simulink model "HIL5DOF_Speedgoat"  (R2026a)
settings: Solver=ode3  StopTime=inf  FixedStep=1/20000
values from neighbouring files (symbols this model uses):
  ems =     [ems11.mat]
  hems =     [Datos_Para_Control_Preciso.mat]
undefined symbols (not defined in the file or in its folder): hems_direct_F_table_H10, hems_direct_gap_bp_H10, hems_direct_I_bp_H10, IO316, IO3xx, m, magnitude, Pull, pull, up, x0, xguid_12, xguid_34, xguid_56, xlev_12, xlev_34, ylev_13, ylev_24, zguid
libraries: speedgoatlib_IO110 x2, aerolibobsolete x1, speedgoatlib_fpga_pwm x1, speedgoatlib_fpga x1
(part 2 of 2)

== system HIL5DOF_Speedgoat/MODELO ELECTROMAGNÉTICO/MODELO ELECTROMAGNETICO EMS/EMS 6 ==
  Tensión Objetivo : Inport
  Airgap : Inport  Port=2
  2-D Lookup Table1 : Lookup_n-D  BreakpointsForDimension1=ems.Airgap  BreakpointsForDimension2=ems.Current  Table=ems.Force_Horizontal  ExtrapMethod=Clip  InternalRulePriority=Speed  RndMeth=Simplest
      settings: InputPortMap=u0,u1
  CIrcuito RL : Subsystem
  Gain : Gain  Gain=1000
  Modelado Temperatura : Subsystem  Commented=through
  Corriente : Outport
  T [ºC] : Outport  Port=2
  Fuerza Horizontal : Outport  Port=3
  wires:
  CIrcuito RL/1(Corriente) -> 2-D Lookup Table1/2, Modelado Temperatura/1(I (A)), Corriente/1
  Tensión Objetivo/1 -> CIrcuito RL/2(Tensión Objetivo)
  Airgap/1 -> Gain/1, CIrcuito RL/1(Airgap)
  Gain/1 -> 2-D Lookup Table1/1
  Modelado Temperatura/1(T [ºC]) -> T [ºC]/1
  2-D Lookup Table1/1 -> Fuerza Horizontal/1

== system HIL5DOF_Speedgoat/MODELO ELECTROMAGNÉTICO/MODELO ELECTROMAGNETICO HEMS/HEMS 1 ==
  Tensión Objetivo : Inport
  Airgap : Inport  Port=2
  2-D Lookup Table1 : Lookup_n-D  Commented=on  BreakpointsForDimension1=hems.Airgap  BreakpointsForDimension2=hems.Current  Table=hems.Force_Horizontal  InternalRulePriority=Speed  RndMeth=Simplest
      settings: InputPortMap=u0,u1
  CIrcuito RL : Subsystem
  Gain : Gain  Gain=1000
  LUT_HEMS_1 : Lookup_n-D  BreakpointsForDimension1=hems_direct_gap_bp_H10  BreakpointsForDimension2=hems_direct_I_bp_H10  Table=hems_direct_F_table_H10  ExtrapMethod=Clip  InternalRulePriority=Speed  RndMeth=Simplest
      settings: InputPortMap=u0,u1
  Fuerza Vertical : Outport
  Corriente : Outport  Port=2
  Fuerza Horizontal : Outport  Port=3
  wires:
  CIrcuito RL/1(Corriente) -> LUT_HEMS_1/2, 2-D Lookup Table1/2, Corriente/1
  Tensión Objetivo/1 -> CIrcuito RL/2(Tensión Objetivo)
  LUT_HEMS_1/1 -> Fuerza Vertical/1
  Airgap/1 -> Gain/1, CIrcuito RL/1(Airgap)
  Gain/1 -> LUT_HEMS_1/1, 2-D Lookup Table1/1
  2-D Lookup Table1/1 -> Fuerza Horizontal/1

== system HIL5DOF_Speedgoat/MODELO ELECTROMAGNÉTICO/MODELO ELECTROMAGNETICO HEMS/HEMS 2 ==
  Tensión Objetivo : Inport
  Airgap : Inport  Port=2
  2-D Lookup Table1 : Lookup_n-D  Commented=on  BreakpointsForDimension1=hems.Airgap  BreakpointsForDimension2=hems.Current  Table=hems.Force_Horizontal  InternalRulePriority=Speed  RndMeth=Simplest
      settings: InputPortMap=u0,u1
  CIrcuito RL : Subsystem
  Gain : Gain  Gain=1000
  LUT_HEMS_1 : Lookup_n-D  BreakpointsForDimension1=hems_direct_gap_bp_H10  BreakpointsForDimension2=hems_direct_I_bp_H10  Table=hems_direct_F_table_H10  ExtrapMethod=Clip  InternalRulePriority=Speed  RndMeth=Simplest
      settings: InputPortMap=u0,u1
  Modelado Temperatura : Subsystem
  Fuerza Vertical : Outport
  Corriente : Outport  Port=2
  T [ºC] : Outport  Port=3
  Fuerza Horizontal : Outport  Port=4
  wires:
  2-D Lookup Table1/1 -> Fuerza Horizontal/1
  Modelado Temperatura/1(T [ºC]) -> T [ºC]/1
  Gain/1 -> LUT_HEMS_1/1, 2-D Lookup Table1/1
  Airgap/1 -> CIrcuito RL/1(Airgap), Gain/1
  LUT_HEMS_1/1 -> Fuerza Vertical/1
  Tensión Objetivo/1 -> CIrcuito RL/2(Tensión Objetivo)
  CIrcuito RL/1(Corriente) -> Corriente/1, LUT_HEMS_1/2, Modelado Temperatura/1(I (A)), 2-D Lookup Table1/2

== system HIL5DOF_Speedgoat/MODELO ELECTROMAGNÉTICO/MODELO ELECTROMAGNETICO HEMS/HEMS 3 ==
  Tensión Objetivo : Inport
  Airgap : Inport  Port=2
  2-D Lookup Table1 : Lookup_n-D  Commented=on  BreakpointsForDimension1=hems.Airgap  BreakpointsForDimension2=hems.Current  Table=hems.Force_Horizontal  InternalRulePriority=Speed  RndMeth=Simplest
      settings: InputPortMap=u0,u1
  CIrcuito RL : Subsystem
  Gain : Gain  Gain=1000
  LUT_HEMS_1 : Lookup_n-D  BreakpointsForDimension1=hems_direct_gap_bp_H10  BreakpointsForDimension2=hems_direct_I_bp_H10  Table=hems_direct_F_table_H10  ExtrapMethod=Clip  InternalRulePriority=Speed  RndMeth=Simplest
      settings: InputPortMap=u0,u1
  Modelado Temperatura : Subsystem
  Fuerza Vertical : Outport
  Corriente : Outport  Port=2
  T [ºC] : Outport  Port=3
  Fuerza Horizontal : Outport  Port=4
  wires:
  CIrcuito RL/1(Corriente) -> LUT_HEMS_1/2, 2-D Lookup Table1/2, Modelado Temperatura/1(I (A)), Corriente/1
  Tensión Objetivo/1 -> CIrcuito RL/2(Tensión Objetivo)
  LUT_HEMS_1/1 -> Fuerza Vertical/1
  Airgap/1 -> Gain/1, CIrcuito RL/1(Airgap)
  Gain/1 -> LUT_HEMS_1/1, 2-D Lookup Table1/1
  Modelado Temperatura/1(T [ºC]) -> T [ºC]/1
  2-D Lookup Table1/1 -> Fuerza Horizontal/1

== system HIL5DOF_Speedgoat/MODELO ELECTROMAGNÉTICO/MODELO ELECTROMAGNETICO HEMS/HEMS 4 ==
  Tensión Objetivo : Inport
  Airgap : Inport  Port=2
  2-D Lookup Table1 : Lookup_n-D  Commented=on  BreakpointsForDimension1=hems.Airgap  BreakpointsForDimension2=hems.Current  Table=hems.Force_Horizontal  InternalRulePriority=Speed  RndMeth=Simplest
      settings: InputPortMap=u0,u1
  CIrcuito RL : Subsystem
  Gain : Gain  Gain=1000
  LUT_HEMS_1 : Lookup_n-D  BreakpointsForDimension1=hems_direct_gap_bp_H10  BreakpointsForDimension2=hems_direct_I_bp_H10  Table=hems_direct_F_table_H10  ExtrapMethod=Clip  InternalRulePriority=Speed  RndMeth=Simplest
      settings: InputPortMap=u0,u1
  Modelado Temperatura : Subsystem
  Fuerza Vertical : Outport
  Corriente : Outport  Port=2
  T [ºC] : Outport  Port=3
  Fuerza Horizontal : Outport  Port=4
  wires:
  2-D Lookup Table1/1 -> Fuerza Horizontal/1
  Modelado Temperatura/1(T [ºC]) -> T [ºC]/1
  Gain/1 -> LUT_HEMS_1/1, 2-D Lookup Table1/1
  Airgap/1 -> CIrcuito RL/1(Airgap), Gain/1
  LUT_HEMS_1/1 -> Fuerza Vertical/1
  Tensión Objetivo/1 -> CIrcuito RL/2(Tensión Objetivo)
  CIrcuito RL/1(Corriente) -> Corriente/1, LUT_HEMS_1/2, Modelado Temperatura/1(I (A)), 2-D Lookup Table1/2

== system HIL5DOF_Speedgoat/MODELO ELECTROMAGNÉTICO/MODELO ELECTROMAGNETICO EMS/EMS 1/CIrcuito RL ==
  Airgap : Inport
  Tensión Objetivo : Inport  Port=2
  Add : Sum  Inputs=+-
  Gain : Gain  Gain=1000
  Inductancia de la Bobina : Lookup_n-D  BreakpointsForDimension1=ems.Airgap  BreakpointsForDimension2=ems.Current(1:54)  Table=ems.Inductance  ExtrapMethod=Clip  InternalRulePriority=Speed  RndMeth=Simplest
      settings: InputPortMap=u0,u1
  Integrator : Integrator
  Product : Product  Inputs=*/
  Product1 : Product  Inputs=/*
  Product2 : Product  Inputs=*/
  Resistencia : Constant  Value=hems.Resistance
  Corriente : Outport
  wires:
  Gain/1 -> Inductancia de la Bobina/1
  Tensión Objetivo/1 -> Product/1
  Product2/1 -> Integrator/1
  Add/1 -> Product2/1
  Integrator/1 -> Add/2, Inductancia de la Bobina/2, Corriente/1
  Airgap/1 -> Gain/1
  Resistencia/1 -> Product/2, Product1/1
  Product/1 -> Add/1
  Product1/1 -> Product2/2
  Inductancia de la Bobina/1 -> Product1/2

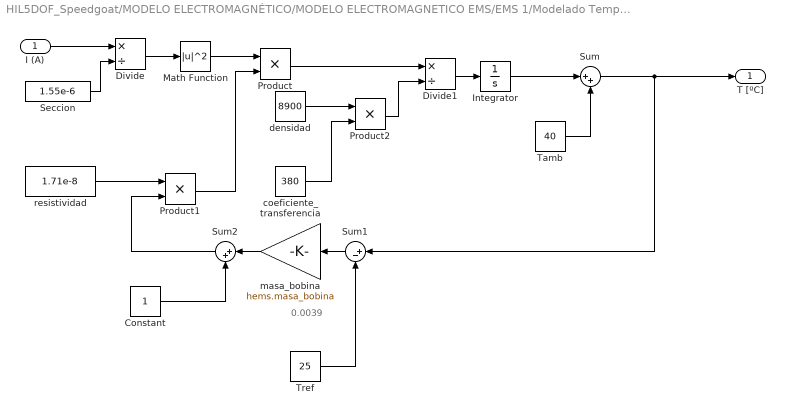
== system HIL5DOF_Speedgoat/MODELO ELECTROMAGNÉTICO/MODELO ELECTROMAGNETICO EMS/EMS 1/Modelado Temperatura ==
  note: 0.0039
  I (A) : Inport
  Constant : Constant
  Divide : Product  Inputs=*/
  Divide1 : Product  Inputs=*/
  Integrator : Integrator
  Math Function : Math  Operator=magnitude^2
  Product : Product
  Product1 : Product
  Product2 : Product
  Seccion : Constant  Value=1.55e-6
  Sum : Sum  Inputs=|++
  Sum1 : Sum  Inputs=|+-
  Sum2 : Sum  Inputs=|++
  Tamb : Constant  Value=40
  Tref : Constant  Value=25
  coeficiente_transferencia : Constant  Value=380
  densidad : Constant  Value=8900
  masa_bobina : Gain  Gain=hems.masa_bobina
  resistividad : Constant  Value=1.71e-8
  T [ºC] : Outport
  wires:
  I (A)/1 -> Divide/1
  Product2/1 -> Divide1/2
  Tref/1 -> Sum1/2
  Tamb/1 -> Sum/2
  Product/1 -> Divide1/1
  masa_bobina/1 -> Sum2/1
  coeficiente_transferencia/1 -> Product2/2
  Sum2/1 -> Product1/2
  Math Function/1 -> Product/1
  Sum/1 -> Sum1/1, T [ºC]/1
  Product1/1 -> Product/2
  Constant/1 -> Sum2/2
  resistividad/1 -> Product1/1
  Divide/1 -> Math Function/1
  densidad/1 -> Product2/1
  Divide1/1 -> Integrator/1
  Seccion/1 -> Divide/2
  Sum1/1 -> masa_bobina/1
  Integrator/1 -> Sum/1

== system HIL5DOF_Speedgoat/MODELO ELECTROMAGNÉTICO/MODELO ELECTROMAGNETICO EMS/EMS 2/CIrcuito RL ==
  Airgap : Inport
  Tensión Objetivo : Inport  Port=2
  Add : Sum  Inputs=+-
  Gain : Gain  Gain=1000
  Inductancia de la Bobina : Lookup_n-D  BreakpointsForDimension1=ems.Airgap  BreakpointsForDimension2=ems.Current(1:54)  Table=ems.Inductance  ExtrapMethod=Clip  InternalRulePriority=Speed  RndMeth=Simplest
      settings: InputPortMap=u0,u1
  Integrator : Integrator
  Product : Product  Inputs=*/
  Product1 : Product  Inputs=/*
  Product2 : Product  Inputs=*/
  Resistencia : Constant  Value=hems.Resistance
  Corriente : Outport
  wires:
  Inductancia de la Bobina/1 -> Product1/2
  Product1/1 -> Product2/2
  Product/1 -> Add/1
  Resistencia/1 -> Product1/1, Product/2
  Airgap/1 -> Gain/1
  Integrator/1 -> Corriente/1, Inductancia de la Bobina/2, Add/2
  Add/1 -> Product2/1
  Product2/1 -> Integrator/1
  Tensión Objetivo/1 -> Product/1
  Gain/1 -> Inductancia de la Bobina/1

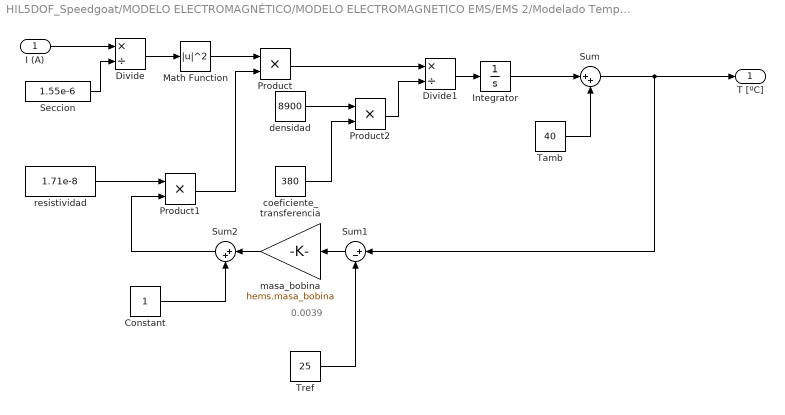
== system HIL5DOF_Speedgoat/MODELO ELECTROMAGNÉTICO/MODELO ELECTROMAGNETICO EMS/EMS 2/Modelado Temperatura ==
  note: 0.0039
  I (A) : Inport
  Constant : Constant
  Divide : Product  Inputs=*/
  Divide1 : Product  Inputs=*/
  Integrator : Integrator
  Math Function : Math  Operator=magnitude^2
  Product : Product
  Product1 : Product
  Product2 : Product
  Seccion : Constant  Value=1.55e-6
  Sum : Sum  Inputs=|++
  Sum1 : Sum  Inputs=|+-
  Sum2 : Sum  Inputs=|++
  Tamb : Constant  Value=40
  Tref : Constant  Value=25
  coeficiente_transferencia : Constant  Value=380
  densidad : Constant  Value=8900
  masa_bobina : Gain  Gain=hems.masa_bobina
  resistividad : Constant  Value=1.71e-8
  T [ºC] : Outport
  wires:
  Integrator/1 -> Sum/1
  Sum1/1 -> masa_bobina/1
  Seccion/1 -> Divide/2
  Divide1/1 -> Integrator/1
  densidad/1 -> Product2/1
  Divide/1 -> Math Function/1
  resistividad/1 -> Product1/1
  Constant/1 -> Sum2/2
  Product1/1 -> Product/2
  Sum/1 -> T [ºC]/1, Sum1/1
  Math Function/1 -> Product/1
  Sum2/1 -> Product1/2
  coeficiente_transferencia/1 -> Product2/2
  masa_bobina/1 -> Sum2/1
  Product/1 -> Divide1/1
  Tamb/1 -> Sum/2
  Tref/1 -> Sum1/2
  Product2/1 -> Divide1/2
  I (A)/1 -> Divide/1

== system HIL5DOF_Speedgoat/MODELO ELECTROMAGNÉTICO/MODELO ELECTROMAGNETICO EMS/EMS 3/CIrcuito RL ==
  Airgap : Inport
  Tensión Objetivo : Inport  Port=2
  Add : Sum  Inputs=+-
  Gain : Gain  Gain=1000
  Inductancia de la Bobina : Lookup_n-D  BreakpointsForDimension1=ems.Airgap  BreakpointsForDimension2=ems.Current(1:54)  Table=ems.Inductance  ExtrapMethod=Clip  InternalRulePriority=Speed  RndMeth=Simplest
      settings: InputPortMap=u0,u1
  Integrator : Integrator
  Product : Product  Inputs=*/
  Product1 : Product  Inputs=/*
  Product2 : Product  Inputs=*/
  Resistencia : Constant  Value=hems.Resistance
  Corriente : Outport
  wires:
  Gain/1 -> Inductancia de la Bobina/1
  Tensión Objetivo/1 -> Product/1
  Product2/1 -> Integrator/1
  Add/1 -> Product2/1
  Integrator/1 -> Add/2, Inductancia de la Bobina/2, Corriente/1
  Airgap/1 -> Gain/1
  Resistencia/1 -> Product/2, Product1/1
  Product/1 -> Add/1
  Product1/1 -> Product2/2
  Inductancia de la Bobina/1 -> Product1/2

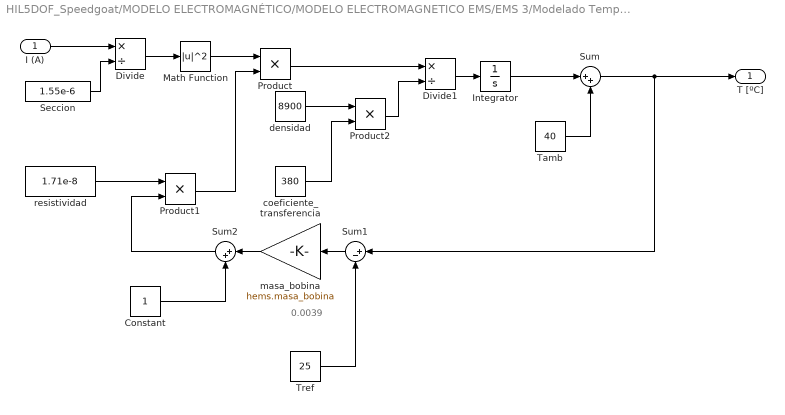
== system HIL5DOF_Speedgoat/MODELO ELECTROMAGNÉTICO/MODELO ELECTROMAGNETICO EMS/EMS 3/Modelado Temperatura ==
  note: 0.0039
  I (A) : Inport
  Constant : Constant
  Divide : Product  Inputs=*/
  Divide1 : Product  Inputs=*/
  Integrator : Integrator
  Math Function : Math  Operator=magnitude^2
  Product : Product
  Product1 : Product
  Product2 : Product
  Seccion : Constant  Value=1.55e-6
  Sum : Sum  Inputs=|++
  Sum1 : Sum  Inputs=|+-
  Sum2 : Sum  Inputs=|++
  Tamb : Constant  Value=40
  Tref : Constant  Value=25
  coeficiente_transferencia : Constant  Value=380
  densidad : Constant  Value=8900
  masa_bobina : Gain  Gain=hems.masa_bobina
  resistividad : Constant  Value=1.71e-8
  T [ºC] : Outport
  wires:
  I (A)/1 -> Divide/1
  Product2/1 -> Divide1/2
  Tref/1 -> Sum1/2
  Tamb/1 -> Sum/2
  Product/1 -> Divide1/1
  masa_bobina/1 -> Sum2/1
  coeficiente_transferencia/1 -> Product2/2
  Sum2/1 -> Product1/2
  Math Function/1 -> Product/1
  Sum/1 -> Sum1/1, T [ºC]/1
  Product1/1 -> Product/2
  Constant/1 -> Sum2/2
  resistividad/1 -> Product1/1
  Divide/1 -> Math Function/1
  densidad/1 -> Product2/1
  Divide1/1 -> Integrator/1
  Seccion/1 -> Divide/2
  Sum1/1 -> masa_bobina/1
  Integrator/1 -> Sum/1

== system HIL5DOF_Speedgoat/MODELO ELECTROMAGNÉTICO/MODELO ELECTROMAGNETICO EMS/EMS 4/CIrcuito RL ==
  Airgap : Inport
  Tensión Objetivo : Inport  Port=2
  Add : Sum  Inputs=+-
  Gain : Gain  Gain=1000
  Inductancia de la Bobina : Lookup_n-D  BreakpointsForDimension1=ems.Airgap  BreakpointsForDimension2=ems.Current(1:54)  Table=ems.Inductance  ExtrapMethod=Clip  InternalRulePriority=Speed  RndMeth=Simplest
      settings: InputPortMap=u0,u1
  Integrator : Integrator
  Product : Product  Inputs=*/
  Product1 : Product  Inputs=/*
  Product2 : Product  Inputs=*/
  Resistencia : Constant  Value=hems.Resistance
  Corriente : Outport
  wires:
  Inductancia de la Bobina/1 -> Product1/2
  Product1/1 -> Product2/2
  Product/1 -> Add/1
  Resistencia/1 -> Product1/1, Product/2
  Airgap/1 -> Gain/1
  Integrator/1 -> Corriente/1, Inductancia de la Bobina/2, Add/2
  Add/1 -> Product2/1
  Product2/1 -> Integrator/1
  Tensión Objetivo/1 -> Product/1
  Gain/1 -> Inductancia de la Bobina/1

== system HIL5DOF_Speedgoat/MODELO ELECTROMAGNÉTICO/MODELO ELECTROMAGNETICO EMS/EMS 4/Modelado Temperatura ==
  note: 0.0039
  I (A) : Inport
  Constant : Constant
  Divide : Product  Inputs=*/
  Divide1 : Product  Inputs=*/
  Integrator : Integrator
  Math Function : Math  Operator=magnitude^2
  Product : Product
  Product1 : Product
  Product2 : Product
  Seccion : Constant  Value=1.55e-6
  Sum : Sum  Inputs=|++
  Sum1 : Sum  Inputs=|+-
  Sum2 : Sum  Inputs=|++
  Tamb : Constant  Value=40
  Tref : Constant  Value=25
  coeficiente_transferencia : Constant  Value=380
  densidad : Constant  Value=8900
  masa_bobina : Gain  Gain=hems.masa_bobina
  resistividad : Constant  Value=1.71e-8
  T [ºC] : Outport
  wires:
  Integrator/1 -> Sum/1
  Sum1/1 -> masa_bobina/1
  Seccion/1 -> Divide/2
  Divide1/1 -> Integrator/1
  densidad/1 -> Product2/1
  Divide/1 -> Math Function/1
  resistividad/1 -> Product1/1
  Constant/1 -> Sum2/2
  Product1/1 -> Product/2
  Sum/1 -> T [ºC]/1, Sum1/1
  Math Function/1 -> Product/1
  Sum2/1 -> Product1/2
  coeficiente_transferencia/1 -> Product2/2
  masa_bobina/1 -> Sum2/1
  Product/1 -> Divide1/1
  Tamb/1 -> Sum/2
  Tref/1 -> Sum1/2
  Product2/1 -> Divide1/2
  I (A)/1 -> Divide/1

== system HIL5DOF_Speedgoat/MODELO ELECTROMAGNÉTICO/MODELO ELECTROMAGNETICO EMS/EMS 5/CIrcuito RL ==
  Airgap : Inport
  Tensión Objetivo : Inport  Port=2
  Add : Sum  Inputs=+-
  Gain : Gain  Gain=1000
  Inductancia de la Bobina : Lookup_n-D  BreakpointsForDimension1=ems.Airgap  BreakpointsForDimension2=ems.Current(1:54)  Table=ems.Inductance  ExtrapMethod=Clip  InternalRulePriority=Speed  RndMeth=Simplest
      settings: InputPortMap=u0,u1
  Integrator : Integrator
  Product : Product  Inputs=*/
  Product1 : Product  Inputs=/*
  Product2 : Product  Inputs=*/
  Resistencia : Constant  Value=hems.Resistance
  Corriente : Outport
  wires:
  Gain/1 -> Inductancia de la Bobina/1
  Tensión Objetivo/1 -> Product/1
  Product2/1 -> Integrator/1
  Add/1 -> Product2/1
  Integrator/1 -> Add/2, Inductancia de la Bobina/2, Corriente/1
  Airgap/1 -> Gain/1
  Resistencia/1 -> Product/2, Product1/1
  Product/1 -> Add/1
  Product1/1 -> Product2/2
  Inductancia de la Bobina/1 -> Product1/2

== system HIL5DOF_Speedgoat/MODELO ELECTROMAGNÉTICO/MODELO ELECTROMAGNETICO EMS/EMS 5/Modelado Temperatura ==
  note: 0.0039
  I (A) : Inport
  Constant : Constant
  Divide : Product  Inputs=*/
  Divide1 : Product  Inputs=*/
  Integrator : Integrator
  Math Function : Math  Operator=magnitude^2
  Product : Product
  Product1 : Product
  Product2 : Product
  Seccion : Constant  Value=1.55e-6
  Sum : Sum  Inputs=|++
  Sum1 : Sum  Inputs=|+-
  Sum2 : Sum  Inputs=|++
  Tamb : Constant  Value=40
  Tref : Constant  Value=25
  coeficiente_transferencia : Constant  Value=380
  densidad : Constant  Value=8900
  masa_bobina : Gain  Gain=hems.masa_bobina
  resistividad : Constant  Value=1.71e-8
  T [ºC] : Outport
  wires:
  I (A)/1 -> Divide/1
  Product2/1 -> Divide1/2
  Tref/1 -> Sum1/2
  Tamb/1 -> Sum/2
  Product/1 -> Divide1/1
  masa_bobina/1 -> Sum2/1
  coeficiente_transferencia/1 -> Product2/2
  Sum2/1 -> Product1/2
  Math Function/1 -> Product/1
  Sum/1 -> Sum1/1, T [ºC]/1
  Product1/1 -> Product/2
  Constant/1 -> Sum2/2
  resistividad/1 -> Product1/1
  Divide/1 -> Math Function/1
  densidad/1 -> Product2/1
  Divide1/1 -> Integrator/1
  Seccion/1 -> Divide/2
  Sum1/1 -> masa_bobina/1
  Integrator/1 -> Sum/1

== system HIL5DOF_Speedgoat/MODELO ELECTROMAGNÉTICO/MODELO ELECTROMAGNETICO EMS/EMS 6/CIrcuito RL ==
  Airgap : Inport
  Tensión Objetivo : Inport  Port=2
  Add : Sum  Inputs=+-
  Gain : Gain  Gain=1000
  Inductancia de la Bobina : Lookup_n-D  BreakpointsForDimension1=ems.Airgap  BreakpointsForDimension2=ems.Current(1:54)  Table=ems.Inductance  ExtrapMethod=Clip  InternalRulePriority=Speed  RndMeth=Simplest
      settings: InputPortMap=u0,u1
  Integrator : Integrator
  Product : Product  Inputs=*/
  Product1 : Product  Inputs=/*
  Product2 : Product  Inputs=*/
  Resistencia : Constant  Value=hems.Resistance
  Corriente : Outport
  wires:
  Inductancia de la Bobina/1 -> Product1/2
  Product1/1 -> Product2/2
  Product/1 -> Add/1
  Resistencia/1 -> Product1/1, Product/2
  Airgap/1 -> Gain/1
  Integrator/1 -> Corriente/1, Inductancia de la Bobina/2, Add/2
  Add/1 -> Product2/1
  Product2/1 -> Integrator/1
  Tensión Objetivo/1 -> Product/1
  Gain/1 -> Inductancia de la Bobina/1

== system HIL5DOF_Speedgoat/MODELO ELECTROMAGNÉTICO/MODELO ELECTROMAGNETICO EMS/EMS 6/Modelado Temperatura ==
  note: 0.0039
  I (A) : Inport
  Constant : Constant
  Divide : Product  Inputs=*/
  Divide1 : Product  Inputs=*/
  Integrator : Integrator
  Math Function : Math  Operator=magnitude^2
  Product : Product
  Product1 : Product
  Product2 : Product
  Seccion : Constant  Value=1.55e-6
  Sum : Sum  Inputs=|++
  Sum1 : Sum  Inputs=|+-
  Sum2 : Sum  Inputs=|++
  Tamb : Constant  Value=40
  Tref : Constant  Value=25
  coeficiente_transferencia : Constant  Value=380
  densidad : Constant  Value=8900
  masa_bobina : Gain  Gain=hems.masa_bobina
  resistividad : Constant  Value=1.71e-8
  T [ºC] : Outport
  wires:
  Integrator/1 -> Sum/1
  Sum1/1 -> masa_bobina/1
  Seccion/1 -> Divide/2
  Divide1/1 -> Integrator/1
  densidad/1 -> Product2/1
  Divide/1 -> Math Function/1
  resistividad/1 -> Product1/1
  Constant/1 -> Sum2/2
  Product1/1 -> Product/2
  Sum/1 -> T [ºC]/1, Sum1/1
  Math Function/1 -> Product/1
  Sum2/1 -> Product1/2
  coeficiente_transferencia/1 -> Product2/2
  masa_bobina/1 -> Sum2/1
  Product/1 -> Divide1/1
  Tamb/1 -> Sum/2
  Tref/1 -> Sum1/2
  Product2/1 -> Divide1/2
  I (A)/1 -> Divide/1

== system HIL5DOF_Speedgoat/MODELO ELECTROMAGNÉTICO/MODELO ELECTROMAGNETICO HEMS/HEMS 1/CIrcuito RL ==
  Airgap : Inport
  Tensión Objetivo : Inport  Port=2
  Add : Sum  Inputs=+-
  Gain : Gain  Gain=1000
  Inductancia de la Bobina : Lookup_n-D  BreakpointsForDimension1=hems.Airgap  BreakpointsForDimension2=hems.Current(1:109)  Table=hems.Inductance  InternalRulePriority=Speed  RndMeth=Simplest
      settings: InputPortMap=u0,u1
  Integrator : Integrator
  Product : Product  Inputs=*/
  Product1 : Product  Inputs=/*
  Product2 : Product  Inputs=*/
  Resistencia : Constant  Value=hems.Resistance
  Corriente : Outport
  wires:
  Inductancia de la Bobina/1 -> Product1/2
  Product1/1 -> Product2/2
  Product/1 -> Add/1
  Resistencia/1 -> Product1/1, Product/2
  Airgap/1 -> Gain/1
  Integrator/1 -> Corriente/1, Inductancia de la Bobina/2, Add/2
  Add/1 -> Product2/1
  Product2/1 -> Integrator/1
  Tensión Objetivo/1 -> Product/1
  Gain/1 -> Inductancia de la Bobina/1

== system HIL5DOF_Speedgoat/MODELO ELECTROMAGNÉTICO/MODELO ELECTROMAGNETICO HEMS/HEMS 2/CIrcuito RL ==
  Airgap : Inport
  Tensión Objetivo : Inport  Port=2
  Add : Sum  Inputs=+-
  Gain : Gain  Gain=1000
  Inductancia de la Bobina : Lookup_n-D  BreakpointsForDimension1=hems.Airgap  BreakpointsForDimension2=hems.Current(1:109)  Table=hems.Inductance  InternalRulePriority=Speed  RndMeth=Simplest
      settings: InputPortMap=u0,u1
  Integrator : Integrator
  Product : Product  Inputs=*/
  Product1 : Product  Inputs=/*
  Product2 : Product  Inputs=*/
  Resistencia : Constant  Value=hems.Resistance
  Corriente : Outport
  wires:
  Gain/1 -> Inductancia de la Bobina/1
  Tensión Objetivo/1 -> Product/1
  Product2/1 -> Integrator/1
  Add/1 -> Product2/1
  Integrator/1 -> Add/2, Inductancia de la Bobina/2, Corriente/1
  Airgap/1 -> Gain/1
  Resistencia/1 -> Product/2, Product1/1
  Product/1 -> Add/1
  Product1/1 -> Product2/2
  Inductancia de la Bobina/1 -> Product1/2

== system HIL5DOF_Speedgoat/MODELO ELECTROMAGNÉTICO/MODELO ELECTROMAGNETICO HEMS/HEMS 2/Modelado Temperatura ==
  note: 0.0039
  I (A) : Inport
  Constant : Constant
  Divide : Product  Inputs=*/
  Divide1 : Product  Inputs=*/
  Integrator : Integrator
  Math Function : Math  Operator=magnitude^2
  Product : Product
  Product1 : Product
  Product2 : Product
  Seccion : Constant  Value=1.55e-6
  Sum : Sum  Inputs=|++
  Sum1 : Sum  Inputs=|+-
  Sum2 : Sum  Inputs=|++
  Tamb : Constant  Value=40
  Tref : Constant  Value=25
  coeficiente_transferencia : Constant  Value=380
  densidad : Constant  Value=8900
  masa_bobina : Gain  Gain=hems.masa_bobina
  resistividad : Constant  Value=1.71e-8
  T [ºC] : Outport
  wires:
  I (A)/1 -> Divide/1
  Product2/1 -> Divide1/2
  Tref/1 -> Sum1/2
  Tamb/1 -> Sum/2
  Product/1 -> Divide1/1
  masa_bobina/1 -> Sum2/1
  coeficiente_transferencia/1 -> Product2/2
  Sum2/1 -> Product1/2
  Math Function/1 -> Product/1
  Sum/1 -> Sum1/1, T [ºC]/1
  Product1/1 -> Product/2
  Constant/1 -> Sum2/2
  resistividad/1 -> Product1/1
  Divide/1 -> Math Function/1
  densidad/1 -> Product2/1
  Divide1/1 -> Integrator/1
  Seccion/1 -> Divide/2
  Sum1/1 -> masa_bobina/1
  Integrator/1 -> Sum/1

== system HIL5DOF_Speedgoat/MODELO ELECTROMAGNÉTICO/MODELO ELECTROMAGNETICO HEMS/HEMS 3/CIrcuito RL ==
  Airgap : Inport
  Tensión Objetivo : Inport  Port=2
  Add : Sum  Inputs=+-
  Gain : Gain  Gain=1000
  Inductancia de la Bobina : Lookup_n-D  BreakpointsForDimension1=hems.Airgap  BreakpointsForDimension2=hems.Current(1:109)  Table=hems.Inductance  InternalRulePriority=Speed  RndMeth=Simplest
      settings: InputPortMap=u0,u1
  Integrator : Integrator
  Product : Product  Inputs=*/
  Product1 : Product  Inputs=/*
  Product2 : Product  Inputs=*/
  Resistencia : Constant  Value=hems.Resistance
  Corriente : Outport
  wires:
  Inductancia de la Bobina/1 -> Product1/2
  Product1/1 -> Product2/2
  Product/1 -> Add/1
  Resistencia/1 -> Product1/1, Product/2
  Airgap/1 -> Gain/1
  Integrator/1 -> Corriente/1, Inductancia de la Bobina/2, Add/2
  Add/1 -> Product2/1
  Product2/1 -> Integrator/1
  Tensión Objetivo/1 -> Product/1
  Gain/1 -> Inductancia de la Bobina/1

== system HIL5DOF_Speedgoat/MODELO ELECTROMAGNÉTICO/MODELO ELECTROMAGNETICO HEMS/HEMS 3/Modelado Temperatura ==
  note: 0.0039
  I (A) : Inport
  Constant : Constant
  Divide : Product  Inputs=*/
  Divide1 : Product  Inputs=*/
  Integrator : Integrator
  Math Function : Math  Operator=magnitude^2
  Product : Product
  Product1 : Product
  Product2 : Product
  Seccion : Constant  Value=1.55e-6
  Sum : Sum  Inputs=|++
  Sum1 : Sum  Inputs=|+-
  Sum2 : Sum  Inputs=|++
  Tamb : Constant  Value=40
  Tref : Constant  Value=25
  coeficiente_transferencia : Constant  Value=380
  densidad : Constant  Value=8900
  masa_bobina : Gain  Gain=hems.masa_bobina
  resistividad : Constant  Value=1.71e-8
  T [ºC] : Outport
  wires:
  Integrator/1 -> Sum/1
  Sum1/1 -> masa_bobina/1
  Seccion/1 -> Divide/2
  Divide1/1 -> Integrator/1
  densidad/1 -> Product2/1
  Divide/1 -> Math Function/1
  resistividad/1 -> Product1/1
  Constant/1 -> Sum2/2
  Product1/1 -> Product/2
  Sum/1 -> T [ºC]/1, Sum1/1
  Math Function/1 -> Product/1
  Sum2/1 -> Product1/2
  coeficiente_transferencia/1 -> Product2/2
  masa_bobina/1 -> Sum2/1
  Product/1 -> Divide1/1
  Tamb/1 -> Sum/2
  Tref/1 -> Sum1/2
  Product2/1 -> Divide1/2
  I (A)/1 -> Divide/1

== system HIL5DOF_Speedgoat/MODELO ELECTROMAGNÉTICO/MODELO ELECTROMAGNETICO HEMS/HEMS 4/CIrcuito RL ==
  Airgap : Inport
  Tensión Objetivo : Inport  Port=2
  Add : Sum  Inputs=+-
  Gain : Gain  Gain=1000
  Inductancia de la Bobina : Lookup_n-D  BreakpointsForDimension1=hems.Airgap  BreakpointsForDimension2=hems.Current(1:109)  Table=hems.Inductance  InternalRulePriority=Speed  RndMeth=Simplest
      settings: InputPortMap=u0,u1
  Integrator : Integrator
  Product : Product  Inputs=*/
  Product1 : Product  Inputs=/*
  Product2 : Product  Inputs=*/
  Resistencia : Constant  Value=hems.Resistance
  Corriente : Outport
  wires:
  Gain/1 -> Inductancia de la Bobina/1
  Tensión Objetivo/1 -> Product/1
  Product2/1 -> Integrator/1
  Add/1 -> Product2/1
  Integrator/1 -> Add/2, Inductancia de la Bobina/2, Corriente/1
  Airgap/1 -> Gain/1
  Resistencia/1 -> Product/2, Product1/1
  Product/1 -> Add/1
  Product1/1 -> Product2/2
  Inductancia de la Bobina/1 -> Product1/2

== system HIL5DOF_Speedgoat/MODELO ELECTROMAGNÉTICO/MODELO ELECTROMAGNETICO HEMS/HEMS 4/Modelado Temperatura ==
  note: 0.0039
  I (A) : Inport
  Constant : Constant
  Divide : Product  Inputs=*/
  Divide1 : Product  Inputs=*/
  Integrator : Integrator
  Math Function : Math  Operator=magnitude^2
  Product : Product
  Product1 : Product
  Product2 : Product
  Seccion : Constant  Value=1.55e-6
  Sum : Sum  Inputs=|++
  Sum1 : Sum  Inputs=|+-
  Sum2 : Sum  Inputs=|++
  Tamb : Constant  Value=40
  Tref : Constant  Value=25
  coeficiente_transferencia : Constant  Value=380
  densidad : Constant  Value=8900
  masa_bobina : Gain  Gain=hems.masa_bobina
  resistividad : Constant  Value=1.71e-8
  T [ºC] : Outport
  wires:
  I (A)/1 -> Divide/1
  Product2/1 -> Divide1/2
  Tref/1 -> Sum1/2
  Tamb/1 -> Sum/2
  Product/1 -> Divide1/1
  masa_bobina/1 -> Sum2/1
  coeficiente_transferencia/1 -> Product2/2
  Sum2/1 -> Product1/2
  Math Function/1 -> Product/1
  Sum/1 -> Sum1/1, T [ºC]/1
  Product1/1 -> Product/2
  Constant/1 -> Sum2/2
  resistividad/1 -> Product1/1
  Divide/1 -> Math Function/1
  densidad/1 -> Product2/1
  Divide1/1 -> Integrator/1
  Seccion/1 -> Divide/2
  Sum1/1 -> masa_bobina/1
  Integrator/1 -> Sum/1

== matlab function HIL5DOF_Speedgoat/POSICION2AIRGAP/Pos2Airgap_AG_LOCALES/MATLAB Function ==
  data: posicion input; airgaps_actuadores output
function airgaps_actuadores = GapsLocales(posicion)
    y = posicion(1);
    z = posicion(2);
    rotx = posicion(3);
    roty = posicion(4);
    rotz = posicion(5);

    x_front = 0.8498;
    x_rear = 0.8752;
    y_left = 0.3055;
    y_right = 0.2395;

    x_h = [ x_front;  x_front; -x_rear; -x_rear];
    y_h = [-y_left;   y_right; -y_left;  y_right];

    g_h = abs(z + y_h.*sin(rotx) - x_h.*sin(roty));

    AG1 = g_h(1);  
    AG2 = g_h(2);  
    AG3 = g_h(3);  
    AG4 = g_h(4);  
    y_Lnom = 0.3592;
    x_ems = 1.276025;
    y_ems = 0.2877;
    z_ems = 0.186484;

    x_e = [ x_ems;  x_ems; 0; 0; -x_ems; -x_ems];
    y_e = [-y_ems;  y_ems; -y_ems; y_ems; -y_ems; y_ems];
    z_e = z_ems*ones(6,1);
    side_e = [-1; 1; -1; 1; -1; 1];
    rail_e = [-y_Lnom; y_Lnom; -y_Lnom; y_Lnom; -y_Lnom; y_Lnom];

    r_y = y_e.*cos(rotz) ...
          + x_e.*sin(rotz) ...
          - z_e.*sin(rotx);

    g_e = side_e.*(rail_e - r_y - y);

    AG5 = g_e(1);   
    AG6 = g_e(2);   
    AG7 = g_e(3);   
    AG8 = g_e(4);   
    AG9 = g_e(5);  
    AG10 = g_e(6);  

    airgaps_actuadores = [AG1; AG2; AG3; AG4; AG5; AG6; AG7; AG8; AG9; AG10];
end

== matlab function HIL5DOF_Speedgoat/POSICION2AIRGAP/Pos2Airgap_SENSOR/MATLAB Function ==
  data: estados input; gaps output
function gaps = Estados_A_Gaps(estados)
    y = estados(1);
    z = estados(2);
    rotx = estados(3);
    roty = estados(4);
    rotz = estados(5);

   
    t_via = 0.015;         
    z_HEMS_CG = -0.032;    
    y_Lnom = 0.277;        

    x_v = [ 1.2536;  1.2560; -1.2814; -1.2790];
    y_v = [-0.3050;  0.2390; -0.3050;  0.2390];
    z_v = [-0.157; -0.157; -0.157; -0.157];

    g_v = -z ...
          - t_via ...
          + z_HEMS_CG ...
          - z_v.*cos(rotx) ...
          + x_v.*sin(roty) ...
          - y_v.*sin(rotx);

    x_l = [ 1.005;  1.005; -1.005; -1.005];
    y_l = [-0.134;  0.134; -0.134;  0.134];
    z_l = [ 0.184;  0.184;  0.184;  0.184];
    side_l = [-1; 1; -1; 1];
    y_rail_l = [-y_Lnom; y_Lnom; -y_Lnom; y_Lnom];

    r_y = y_l.*cos(rotz) ...
          + x_l.*sin(rotz) ...
          - z_l.*sin(rotx);

    g_l = side_l.*(y_rail_l - r_y - y);

    AG1 = g_v(1);  
    AG2 = g_v(2);  
    AG3 = g_v(3);  
    AG4 = g_v(4);  
    AG5 = g_l(1);  
    AG6 = g_l(2); 
    AG7 = g_l(3);  
    AG8 = g_l(4);  

    gaps = [AG1; AG2; AG3; AG4; AG5; AG6; AG7; AG8];
end

== matlab function HIL5DOF_Speedgoat/Duty to Voltage/PWM pairs to Vctrl ==
  data: Duty input; Voltage output; Flag input
function Voltage = fcn(Duty, Flag)
persistent lastVoltage
if isempty(lastVoltage)
    lastVoltage = zeros(10,1);
end
Voltage = lastVoltage;
for k = 1:10
    a = 2*k - 1;
    b = 2*k;
    if Flag(a) ~= 0 && Flag(b) ~= 0
        lastVoltage(k) = 400.0 * (double(Duty(b)) - double(Duty(a)));
    end
    Voltage(k) = lastVoltage(k);
end
end

== matlab function HIL5DOF_Speedgoat/DINÁMICA DEL SISTEMA/Fuerzas y momentos Eje Z/MATLAB Function1 ==
  data: posicion input; Error_fuerza input; fuerza_resultante output; m input
function fuerza_resultante = fcn(posicion, Error_fuerza, m)
    if posicion >= 0.025
        if Error_fuerza >= 0
            fuerza_resultante = 0;
        else
            fuerza_resultante = Error_fuerza;
        end
    else
        fuerza_resultante = Error_fuerza;
    end
end
